simulink model "HeatX2DRect_ADI"  (R2015a)
settings: Solver=FixedStepDiscrete  StartTime=0.0  StopTime=tsim  FixedStep=dt  RelTol=1e-3
values from neighbouring files (symbols this model uses):
  Cp2d = Cp*ones(length(y0),length(x))    [run_HeatX2DRect.m]
  hb = 0.05    [run_HeatX2DRect.m]
  hl = 0.05    [run_HeatX2DRect.m]
  hr = 0.05    [run_HeatX2DRect.m]
  ht = 0.05    [run_HeatX2DRect.m]
  k2d = k*ones(length(y0),length(x))    [run_HeatX2DRect.m]
  m = length(y0)    [run_HeatX2DRect.m]
  n = length(x)    [run_HeatX2DRect.m]
  rho2d = rho*ones(length(y0),length(x))    [run_HeatX2DRect.m]
  Tb = 850    [run_HeatX2DRect.m]
  Tl = 850    [run_HeatX2DRect.m]
  Tr = 850    [run_HeatX2DRect.m]
  Tt = 850    [run_HeatX2DRect.m]
libraries: lib_Conduction_2DCondADI x1
settings Model: Creator=jlkratz  LastModifiedBy=jlkratz

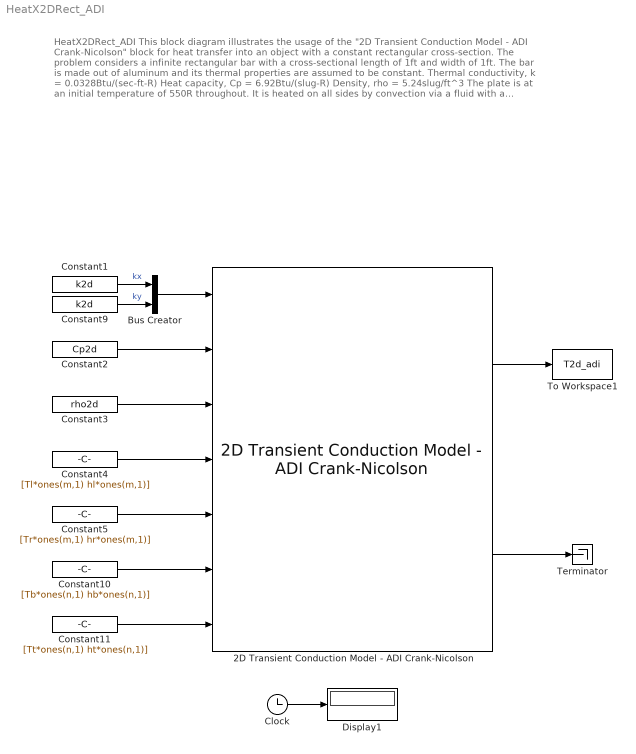
== system HeatX2DRect_ADI ==
  note: HeatX2DRect_ADI
      |
      | This block diagram illustrates the usage of the "2D Transient Conduction Model - ADI Crank-Nicolson" block
      | for heat transfer into an object with a constant rectangular cross-section.
      |
      | The problem considers a infinite rectangular bar with a cross-sectional length of 1ft and width of 1ft. The bar is made
      | out of aluminum and its thermal properties are assumed to be constant.
      | Thermal conductivity, k = 0.0328Btu/(sec-ft-R)
      | Heat capacity, Cp = 6.92Btu/(slug-R)
      | Density, rho = 5.24slug/ft^3
      | The plate is at an initial temperature of 550R throughout. It is heated on all sides by convection via a fluid with a
      | temperature of 850R and a heat transfer coefficient of 0.05Btu/(sec-ft^2-R)
  2D Transient Conduction Model - ADI Crank-Nicolson : lib_Conduction_2DCondADI/2D Transient Conduction Model - ADI Crank-Nicolson  T0_M=T02d  dt_M=dt  x_M=x  y_M=y0  shape_M=Planar in both directions  convL_M=on  radL_M=off  condL_M=off  convR_M=on  radR_M=off  condR_M=off  convB_M=on  radB_M=off  condB_M=off  convT_M=on  radT_M=off  condT_M=off  BN_M=double(gcb)
  Bus Creator : BusCreator  Inputs=2
  Clock : Clock
  Constant1 : Constant  Value=k2d
  Constant10 : Constant  Value=[Tb*ones(n,1) hb*ones(n,1)]
  Constant11 : Constant  Value=[Tt*ones(n,1) ht*ones(n,1)]
  Constant2 : Constant  Value=Cp2d
  Constant3 : Constant  Value=rho2d
  Constant4 : Constant  Value=[Tl*ones(m,1) hl*ones(m,1)]
  Constant5 : Constant  Value=[Tr*ones(m,1) hr*ones(m,1)]
  Constant9 : Constant  Value=k2d
  Display1 : Display
  Terminator : Terminator
  To Workspace1 : ToWorkspace  VariableName=T2d_adi  SaveFormat=Timeseries  SampleTime=-1
  wires:
  Constant1/1 -> Bus Creator/1  "kx"
  Constant9/1 -> Bus Creator/2  "ky"
  Bus Creator/1 -> 2D Transient Conduction Model - ADI Crank-Nicolson/1
  Constant2/1 -> 2D Transient Conduction Model - ADI Crank-Nicolson/2
  Constant3/1 -> 2D Transient Conduction Model - ADI Crank-Nicolson/3
  Constant11/1 -> 2D Transient Conduction Model - ADI Crank-Nicolson/7
  Constant10/1 -> 2D Transient Conduction Model - ADI Crank-Nicolson/6
  2D Transient Conduction Model - ADI Crank-Nicolson/1 -> To Workspace1/1
  2D Transient Conduction Model - ADI Crank-Nicolson/2 -> Terminator/1
  Constant4/1 -> 2D Transient Conduction Model - ADI Crank-Nicolson/4
  Constant5/1 -> 2D Transient Conduction Model - ADI Crank-Nicolson/5
  Clock/1 -> Display1/1
